simulink model "window_discriminator_3"  (R2018a)
settings: Solver=FixedStepAuto  StartTime=0.0  StopTime=6  RelTol=1e-3
PreLoadFcn:
  | load('alberto_data.mat')
model workspace (MAT data in the model file):
  dac_stop_max = 3
  threshold = [-50; -300]
  win_start = [0; 0]
  win_stop = [3; 3]
libraries: simulink x7
settings Model: Creator=stefanobuccelli  LastModifiedBy=stefanobuccelli

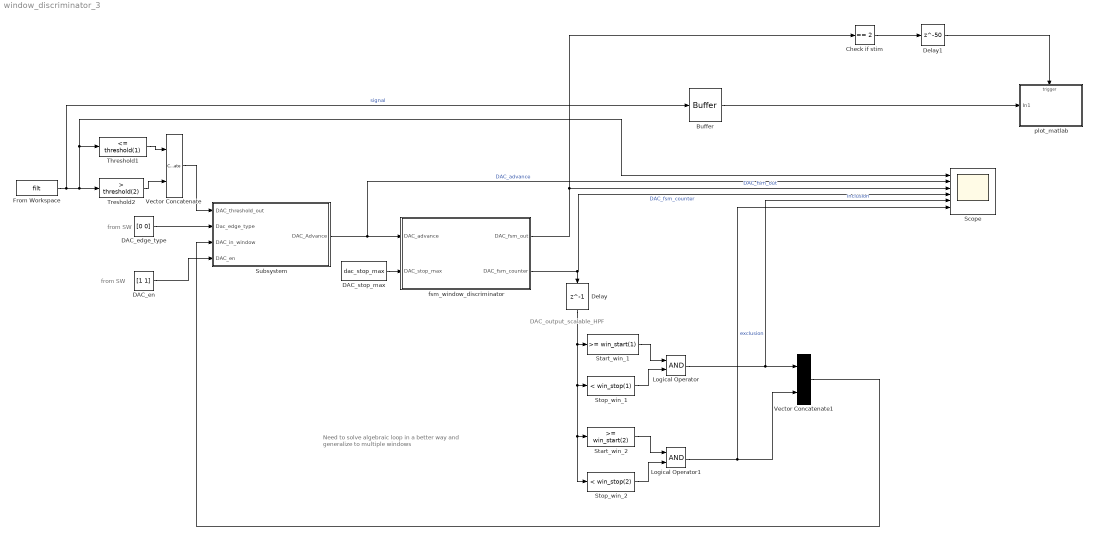
== system window_discriminator_3 ==
  note: Need to solve algebraic loop in a better way and generalize to multiple windows
  note: DAC_output_scalable_HPF
  note: from SW
  note: from SW
  Buffer : Buffer  N=100  V=99  OutputFrames=off
  Check if stim : simulink/Logic and Bit Operations/Compare To Constant  relop===  const=2  OutDataTypeStr=boolean
  DAC_edge_type : Constant  Value=[0 0]  OutDataTypeStr=boolean
  DAC_en : Constant  Value=[1 1]  OutDataTypeStr=boolean
  DAC_stop_max : Constant  Value=dac_stop_max  OutDataTypeStr=double
  Delay : Delay  DelayLength=1
  Delay1 : Delay  DelayLength=50
  From Workspace : FromWorkspace  VariableName=filt  SampleTime=1/25000
  Logical Operator : Logic  AllPortsSameDT=off  OutDataTypeStr=boolean
  Logical Operator1 : Logic  AllPortsSameDT=off  OutDataTypeStr=boolean
  Scope : Scope  NumInputPorts=6
  Start_win_1 : simulink/Logic and Bit Operations/Compare To Constant  relop=>=  const=win_start(1)  OutDataTypeStr=boolean
  Start_win_2 : simulink/Logic and Bit Operations/Compare To Constant  relop=>=  const=win_start(2)  OutDataTypeStr=boolean
  Stop_win_1 : simulink/Logic and Bit Operations/Compare To Constant  relop=<  const=win_stop(1)  OutDataTypeStr=boolean
  Stop_win_2 : simulink/Logic and Bit Operations/Compare To Constant  relop=<  const=win_stop(2)  OutDataTypeStr=boolean
  Subsystem : Subsystem
  Threshold1 : simulink/Logic and Bit Operations/Compare To Constant  relop=<=  const=threshold(1)  OutDataTypeStr=boolean
  Treshold2 : simulink/Logic and Bit Operations/Compare To Constant  relop=>  const=threshold(2)  OutDataTypeStr=boolean
  Vector Concatenate : Concatenate
  Vector Concatenate1 : Concatenate
  fsm_window_discriminator : Stateflow chart  TreatAsAtomicUnit=on
  plot_matlab : Subsystem
  wires:
  fsm_window_discriminator/1(DAC_fsm_out) -> Check if stim/1, Scope/3  "DAC_fsm_out"
  From Workspace/1 -> Buffer/1, Treshold2/1, Threshold1/1, Scope/1  "signal"
  Subsystem/1(DAC_Advance) -> Scope/2, fsm_window_discriminator/1(DAC_advance)  "DAC_advance"
  DAC_edge_type/1 -> Subsystem/2(Dac_edge_type)
  Logical Operator/1 -> Scope/5, Vector Concatenate1/1  "inclusion"
  DAC_en/1 -> Subsystem/4(DAC_en)
  DAC_stop_max/1 -> fsm_window_discriminator/2(DAC_stop_max)
  fsm_window_discriminator/2(DAC_fsm_counter) -> Delay/1, Scope/4  "DAC_fsm_counter"
  Start_win_1/1 -> Logical Operator/1
  Stop_win_1/1 -> Logical Operator/2
  Logical Operator1/1 -> Scope/6, Vector Concatenate1/2  "exclusion"
  Start_win_2/1 -> Logical Operator1/1
  Stop_win_2/1 -> Logical Operator1/2
  Threshold1/1 -> Vector Concatenate/1
  Treshold2/1 -> Vector Concatenate/2
  Vector Concatenate/1 -> Subsystem/1(DAC_threshold_out)
  Vector Concatenate1/1 -> Subsystem/3(DAC_in_window)
  Check if stim/1 -> Delay1/1
  Buffer/1 -> plot_matlab/1(In1)
  Delay1/1 -> plot_matlab/Trigger
  Delay/1 -> Start_win_2/1, Stop_win_2/1, Stop_win_1/1, Start_win_1/1

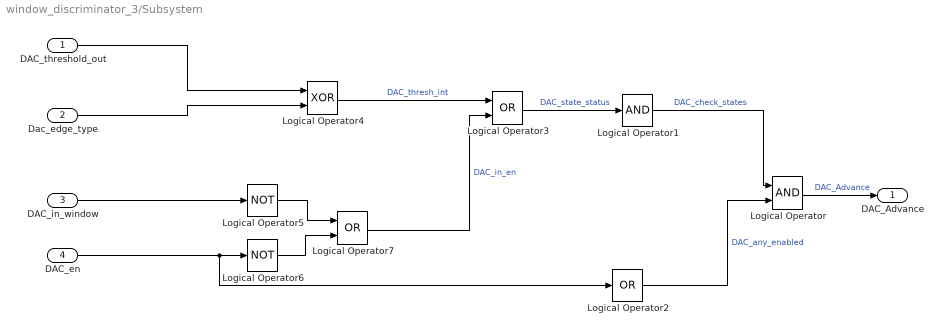
== system window_discriminator_3/Subsystem ==
  DAC_threshold_out : Inport
  Dac_edge_type : Inport  Port=2
  DAC_in_window : Inport  Port=3
  DAC_en : Inport  Port=4
  Logical Operator : Logic  AllPortsSameDT=off  OutDataTypeStr=boolean
  Logical Operator1 : Logic  Inputs=1  AllPortsSameDT=off  OutDataTypeStr=boolean
  Logical Operator2 : Logic  Operator=OR  Inputs=1  AllPortsSameDT=off  OutDataTypeStr=boolean
  Logical Operator3 : Logic  Operator=OR  AllPortsSameDT=off  OutDataTypeStr=boolean
  Logical Operator4 : Logic  Operator=XOR  AllPortsSameDT=off  OutDataTypeStr=boolean
  Logical Operator5 : Logic  Operator=NOT  Inputs=1  AllPortsSameDT=off  OutDataTypeStr=boolean
  Logical Operator6 : Logic  Operator=NOT  Inputs=1  AllPortsSameDT=off  OutDataTypeStr=boolean
  Logical Operator7 : Logic  Operator=OR  AllPortsSameDT=off  OutDataTypeStr=boolean
  DAC_Advance : Outport
  wires:
  Logical Operator/1 -> DAC_Advance/1  "DAC_Advance"
  Logical Operator2/1 -> Logical Operator/2  "DAC_any_enabled"
  Logical Operator1/1 -> Logical Operator/1  "DAC_check_states"
  Logical Operator4/1 -> Logical Operator3/1  "DAC_thresh_int"
  Logical Operator5/1 -> Logical Operator7/1
  DAC_threshold_out/1 -> Logical Operator4/1
  DAC_en/1 -> Logical Operator2/1, Logical Operator6/1
  Logical Operator3/1 -> Logical Operator1/1  "DAC_state_status"
  Logical Operator6/1 -> Logical Operator7/2
  Logical Operator7/1 -> Logical Operator3/2  "DAC_in_en"
  Dac_edge_type/1 -> Logical Operator4/2
  DAC_in_window/1 -> Logical Operator5/1

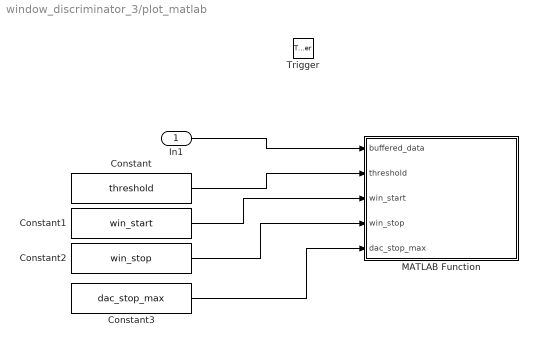
== system window_discriminator_3/plot_matlab ==
  In1 : Inport
  Trigger : TriggerPort  VariantControl=Variant  PortDimensions=1
  Constant : Constant  Value=threshold
  Constant1 : Constant  Value=win_start
  Constant2 : Constant  Value=win_stop
  Constant3 : Constant  Value=dac_stop_max
  MATLAB Function : MATLAB Function  TreatAsAtomicUnit=on
  wires:
  In1/1 -> MATLAB Function/1(buffered_data)
  Constant1/1 -> MATLAB Function/3(win_start)
  Constant/1 -> MATLAB Function/2(threshold)
  Constant2/1 -> MATLAB Function/4(win_stop)
  Constant3/1 -> MATLAB Function/5(dac_stop_max)

== matlab function window_discriminator_3/plot_matlab/MATLAB Function ==
  data: buffered_data input; threshold input; win_start input; win_stop input; dac_stop_max input
function  fcn(buffered_data,threshold,win_start,win_stop,dac_stop_max)
shift=length(buffered_data)/2;
figure(1)
plot((1:length(buffered_data))-shift,buffered_data,'k')
hold on
for curr_DAC=1:length(threshold)
    plot([win_start(curr_DAC):win_stop(curr_DAC)-1]-dac_stop_max,repmat(threshold(curr_DAC),1,length(win_start(curr_DAC):win_stop(curr_DAC)-1)),'b')
end
% the -1 in the start-stop win position is due to the delay (I guess XD)

== stateflow chart window_discriminator_3/fsm_window_discriminator ==
  state IDLE
    entry: DAC_fsm_out=0
    DAC_fsm_counter=0
  state TRACK
    entry: DAC_fsm_out=1
    DAC_fsm_counter=DAC_fsm_counter+1
  state STIM
    entry: DAC_fsm_out=2
    DAC_fsm_counter=0
  (default) -> IDLE
  STIM -> IDLE
  TRACK -> IDLE [order 2] : [~DAC_advance]
  IDLE -> TRACK : [DAC_advance]
  TRACK -> TRACK [order 3] : [DAC_fsm_counter~=DAC_stop_max]
  TRACK -> STIM [order 1] : [DAC_fsm_counter==DAC_stop_max]
  data: DAC_advance input; DAC_fsm_out output double; DAC_stop_max input; DAC_fsm_counter output double
